simulink model "controllo_adattativo"  (R2022b)
settings: Solver=VariableStepAuto  StartTime=0.0  StopTime=40  RelTol=1e-3
values from neighbouring files (symbols this model uses):
  K_pi = diag([100 100 100 100 100 100 100 100 100 100 100 100 0.1 100 100 100])    [controllo_script.m]
  Kd_ad = diag([250 250 250 250])    [controllo_script.m]
  Lambda = diag([50 50 50 50])    [controllo_script.m]
  pi_0 = [m1; I1(3,3); Im1(3,3); Fm(1,1); m2; I2(3,3); Im2(3,3); Fm(2,2); m3; 0; Im3(3,3); Fm(3,3); 0; I4(3,3); Im4(3,3); Fm(4,4)]    [controllo_script.m]
  T = T_A * T_B    [DH_dinamica.m]    (also in traiettoria_script.m = 0.001)
  theta1_0 = pi/2 - angolo    [CLIK_script.m]
  theta2_0 = 2*angolo    [CLIK_script.m]
undefined symbols (not defined in the file or in its folder): DiscIntNeverNeededParam
settings Model: Creator=Principale  LastModifiedBy=Michele
settings DataIOCC: ReturnWorkspaceOutputs=off

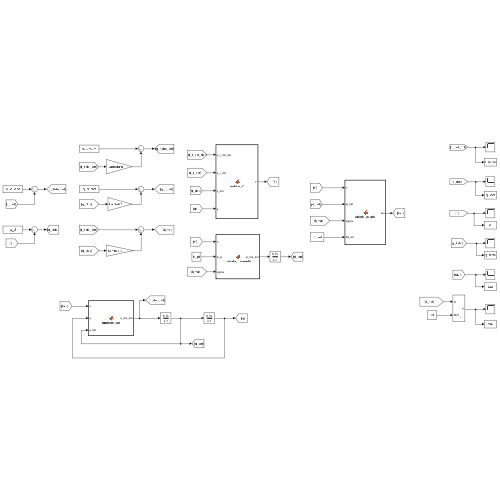
[thumbnail: Simulink's stored preview of the top-level diagram]
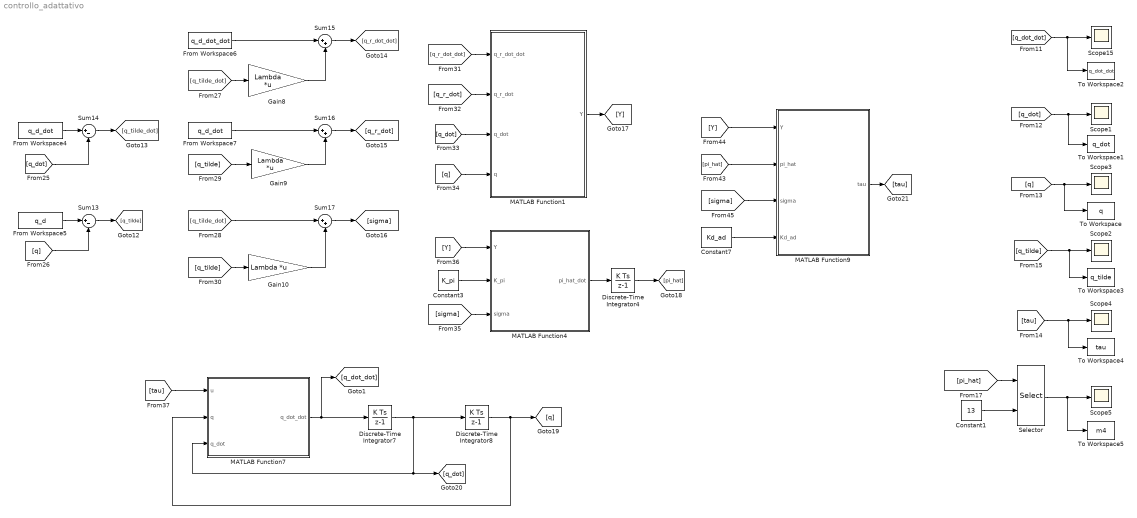
== system controllo_adattativo ==
  Constant1 : Constant  Value=13
  Constant3 : Constant  Value=K_pi  SampleTime=T
  Constant7 : Constant  Value=Kd_ad  SampleTime=T
  Discrete-Time Integrator4 : DiscreteIntegrator  InitialCondition=pi_0  SampleTime=T  ICPrevOutput=DiscIntNeverNeededParam  ICPrevScaledInput=DiscIntNeverNeededParam
  Discrete-Time Integrator7 : DiscreteIntegrator  InitialCondition=[0 0 0 0]'  SampleTime=-1  ICPrevOutput=DiscIntNeverNeededParam  ICPrevScaledInput=DiscIntNeverNeededParam
  Discrete-Time Integrator8 : DiscreteIntegrator  InitialCondition=[theta1_0 theta2_0 -0.25 0]'  SampleTime=-1  ICPrevOutput=DiscIntNeverNeededParam  ICPrevScaledInput=DiscIntNeverNeededParam
  From Workspace4 : FromWorkspace  VariableName=q_d_dot  SampleTime=T
  From Workspace5 : FromWorkspace  VariableName=q_d  SampleTime=T
  From Workspace6 : FromWorkspace  VariableName=q_d_dot_dot  SampleTime=T
  From Workspace7 : FromWorkspace  VariableName=q_d_dot  SampleTime=T
  Gain10 : Gain  Gain=Lambda  Multiplication=Matrix(K*u)
  Gain8 : Gain  Gain=Lambda  Multiplication=Matrix(K*u)
  Gain9 : Gain  Gain=Lambda  Multiplication=Matrix(K*u)
  MATLAB Function1 : MATLAB Function  TreatAsAtomicUnit=on
  MATLAB Function4 : MATLAB Function  TreatAsAtomicUnit=on
  MATLAB Function7 : MATLAB Function  TreatAsAtomicUnit=on
  MATLAB Function9 : MATLAB Function  TreatAsAtomicUnit=on
  Scope{1..5,15} (6 alike) : Scope
  Selector : Selector  InputPortWidth=16  IndexOptions=Index vector (port)  Indices=[1 3]  OutputSizes=1
  Sum13 : Sum  Inputs=|+-
  Sum14 : Sum  Inputs=|+-
  Sum15 : Sum  Inputs=|++
  Sum16 : Sum  Inputs=|++
  Sum17 : Sum  Inputs=|++
  To Workspace : ToWorkspace  VariableName=q  SaveFormat=Structure With Time  SampleTime=-1
  To Workspace1 : ToWorkspace  VariableName=q_dot  SaveFormat=Structure With Time  SampleTime=-1
  To Workspace2 : ToWorkspace  VariableName=q_dot_dot  SaveFormat=Structure With Time  SampleTime=-1
  To Workspace3 : ToWorkspace  VariableName=q_tilde  SaveFormat=Structure With Time  SampleTime=-1
  To Workspace4 : ToWorkspace  VariableName=tau  SaveFormat=Structure With Time  SampleTime=-1
  To Workspace5 : ToWorkspace  VariableName=m4  SaveFormat=Structure With Time  SampleTime=-1
  wires:
  From Workspace4/1 -> Sum14/1
  [q_dot] -> Sum14/2
  From Workspace5/1 -> Sum13/1
  [q] -> Sum13/2
  Sum13/1 -> [q_tilde]
  Sum14/1 -> [q_tilde_dot]
  [q_tilde_dot] -> Gain8/1
  From Workspace6/1 -> Sum15/1
  Gain8/1 -> Sum15/2
  Sum15/1 -> [q_r_dot_dot]
  Sum16/1 -> [q_r_dot]
  Gain9/1 -> Sum16/2
  [q_tilde] -> Gain9/1
  From Workspace7/1 -> Sum16/1
  [q_tilde] -> Gain10/1
  [q_tilde_dot] -> Sum17/1
  Gain10/1 -> Sum17/2
  Sum17/1 -> [sigma]
  [q_r_dot_dot] -> MATLAB Function1/1(q_r_dot_dot)
  [q_r_dot] -> MATLAB Function1/2(q_r_dot)
  [q_dot] -> MATLAB Function1/3(q_dot)
  [q] -> MATLAB Function1/4(q)
  Constant3/1 -> MATLAB Function4/2(K_pi)
  [sigma] -> MATLAB Function4/3(sigma)
  MATLAB Function4/1(pi_hat_dot) -> Discrete-Time Integrator4/1
  MATLAB Function1/1(Y) -> [Y]
  [Y] -> MATLAB Function4/1(Y)
  Discrete-Time Integrator4/1 -> [pi_hat]
  Constant7/1 -> MATLAB Function9/4(Kd_ad)
  [sigma] -> MATLAB Function9/3(sigma)
  [Y] -> MATLAB Function9/1(Y)
  MATLAB Function9/1(tau) -> [tau]
  [pi_hat] -> MATLAB Function9/2(pi_hat)
  Discrete-Time Integrator8/1 -> [q], MATLAB Function7/2(q)
  MATLAB Function7/1(q_dot_dot) -> [q_dot_dot], Discrete-Time Integrator7/1
  Discrete-Time Integrator7/1 -> Discrete-Time Integrator8/1, [q_dot], MATLAB Function7/3(q_dot)
  [tau] -> MATLAB Function7/1(u)
  Selector/1 -> To Workspace5/1, Scope5/1
  [q_dot_dot] -> To Workspace2/1, Scope15/1
  [q_dot] -> To Workspace1/1, Scope1/1
  [q] -> To Workspace/1, Scope3/1
  [q_tilde] -> To Workspace3/1, Scope2/1
  [tau] -> To Workspace4/1, Scope4/1
  [pi_hat] -> Selector/1
  Constant1/1 -> Selector/2

== matlab function controllo_adattativo/MATLAB Function1 ==
  data: q_r_dot_dot input; Y output; q_r_dot input; q_dot input; q input
function Y = matrice_Y(q_r_dot_dot, q_r_dot, q_dot, q)

    qrdd_1 = q_r_dot_dot(1);
    qrdd_2 = q_r_dot_dot(2);
    qrdd_3 = q_r_dot_dot(3);
    qrdd_4 = q_r_dot_dot(4);
    
    qrd_1 = q_r_dot(1);
    qrd_2 = q_r_dot(2);
    qrd_3 = q_r_dot(3);
    qrd_4 = q_r_dot(4);
    
    q1 = q(1);
    q2 = q(2);
    q3 = q(3);
    q4 = q(4);
    
    qdot_1 = q_dot(1);
    qdot_2 = q_dot(2);
    qdot_3 = q_dot(3);
    qdot_4 = q_dot(4);

    Y = [qrdd_1/16, qrdd_1, qrdd_1, qrd_1, qrdd_1*(cos(q2)/4 + 5/16) - qrd_2*((conj(qdot_1)*sin(q2))/8 + (conj(qdot_2)*sin(q2))/8) + qrdd_2*(cos(q2)/8 + 1/16) - (qrd_1*conj(qdot_2)*sin(q2))/8, qrdd_1 + qrdd_2, qrdd_1 + qrdd_2,     0, 0, 0,         qrdd_1 + qrdd_2 + 50*qrdd_3,          0, qrdd_1*(cos(q2)/2 + 1/2) - qrd_2*((conj(qdot_1)*sin(q2))/4 + (conj(qdot_2)*sin(q2))/4) + qrdd_2*(cos(q2)/4 + 1/4) - (qrd_1*conj(qdot_2)*sin(q2))/4, qrdd_1 + qrdd_2 + qrdd_4,        qrdd_1 + qrdd_2 + 20*qrdd_4,         0;
            0,      0,      0,     0,                                                                               qrdd_2/16 + qrdd_1*(cos(q2)/8 + 1/16) + (qrd_1*conj(qdot_1)*sin(q2))/8, qrdd_1 + qrdd_2, qrdd_1 + qrdd_2, qrd_2, 0, 0,         qrdd_1 + qrdd_2 + 50*qrdd_3,          0,                                                                               qrdd_2/4 + qrdd_1*(cos(q2)/4 + 1/4) + (qrd_1*conj(qdot_1)*sin(q2))/4, qrdd_1 + qrdd_2 + qrdd_4,        qrdd_1 + qrdd_2 + 20*qrdd_4,         0;
            0,      0,      0,     0,                                                                                                                                                    0,               0,               0,     0, 0, 0, 50*qrdd_1 + 50*qrdd_2 + 2500*qrdd_3, 2500*qrd_3,                                                                                                                                   qrdd_3 + 981/100,                        0,                                  0,         0;
            0,      0,      0,     0,                                                                                                                                                 0,               0,               0,     0, 0, 0,                                   0,          0,                                                                                                                                                  0, qrdd_1 + qrdd_2 + qrdd_4, 20*qrdd_1 + 20*qrdd_2 + 400*qrdd_4, 400*qrd_4];

end

== matlab function controllo_adattativo/MATLAB Function4 ==
  data: Y input; K_pi input; pi_hat_dot output; sigma input
function pi_hat_dot = derivata_parametri(Y,K_pi,sigma)
    pi_hat_dot = K_pi\(Y'*sigma);
end

== matlab function controllo_adattativo/MATLAB Function7 ==
  data: u input; q input; q_dot_dot output; q_dot input
function q_dot_dot = manipolatore(u, q, q_dot)

    q1 = q(1);
    q2 = q(2);
    q3 = q(3);
    q4 = q(4);
    
    qdot_1 = q_dot(1);
    qdot_2 = q_dot(2);
    qdot_3 = q_dot(3);
    qdot_4 = q_dot(4);
    
    % B
    B = [12*cos(q2) + 11763/500, 6*cos(q2) + 4883/500,  1/4, 51/50;
         6*cos(q2) + 4883/500,             4883/500,  1/4, 51/50;
                       1/4,                  1/4, 53/2,     0;
                     51/50,                51/50,    0,   7/5];
    
    
    % n
    
    n = [conj(qdot_1)/20000 - 6*conj(qdot_2)^2*sin(q2) - 12*conj(qdot_1)*conj(qdot_2)*sin(q2);
        conj(qdot_2)/20000 + 6*conj(qdot_1)^2*sin(q2);
        25*conj(qdot_3) + 6867/50;
        2*conj(qdot_4)];
    
    q_dot_dot = B\(u-n);
end

== matlab function controllo_adattativo/MATLAB Function9 ==
  data: Y input; tau output; pi_hat input; sigma input; Kd_ad input
function tau = calcolo_coppie(Y,pi_hat,sigma,Kd_ad)
    tau = Y*pi_hat + Kd_ad*sigma;
end
